simulink model "LQI"  (R2017a)
settings: Solver=VariableStepAuto  StartTime=0.0  StopTime=10.0  RelTol=1e-3
values from neighbouring files (symbols this model uses):
  u_0 = R*x3_0    [general.m]    (also in general_lqi.m)
  x_0 = [x1_0 x2_0 x3_0]    [general.m]    (also in general_lqi.m)
undefined symbols (not defined in the file or in its folder): K
settings Model: Creator=Daniel  LastModifiedBy=Daniel

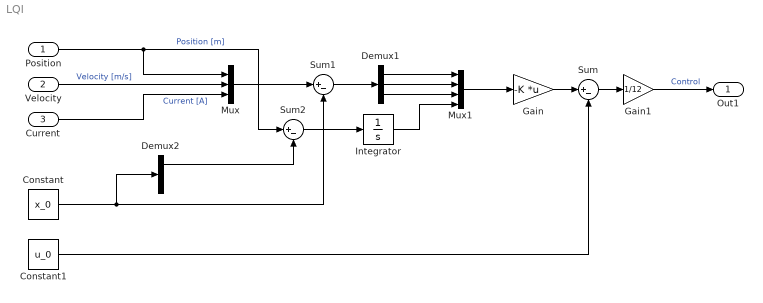
== system LQI ==
  Position : Inport
  Velocity : Inport  Port=2
  Current : Inport  Port=3
  Constant : Constant  Value=x_0
  Constant1 : Constant  Value=u_0
  Demux1 : Demux  Outputs=3
  Demux2 : Demux  Outputs=3
  Gain : Gain  Gain=-K  Multiplication=Matrix(K*u) (u vector)
  Gain1 : Gain  Gain=1/12
  Integrator : Integrator
  Mux : Mux  Inputs=3
  Mux1 : Mux
  Sum : Sum  Inputs=|+-
  Sum1 : Sum  Inputs=|+-
  Sum2 : Sum  Inputs=|+-
  Out1 : Outport
  wires:
  Sum1/1 -> Demux1/1
  Demux1/2 -> Mux1/2
  Demux1/3 -> Mux1/3
  Demux1/1 -> Mux1/1
  Demux2/1 -> Sum2/2
  Integrator/1 -> Mux1/4
  Mux/1 -> Sum1/1
  Mux1/1 -> Gain/1
  Velocity/1 -> Mux/2  "Velocity [m/s]"
  Constant/1 -> Sum1/2, Demux2/1
  Sum2/1 -> Integrator/1
  Position/1 -> Mux/1, Sum2/1  "Position [m]"
  Sum/1 -> Gain1/1
  Constant1/1 -> Sum/2
  Gain1/1 -> Out1/1  "Control"
  Gain/1 -> Sum/1
  Current/1 -> Mux/3  "Current [A]"
